simulink model "random_a"  (Simulink 7.1)
settings: Solver=ode45  StartTime=0.0  StopTime=60.0  RelTol=1e-3
settings Model: Creator=Usuario  LastModifiedBy=Usuario  BufferReuse=off
settings OptimizationCC: OptimizeBlockIOStorage=off  BufferReuse=off  ExpressionFolding=off  LocalBlockOutputs=off

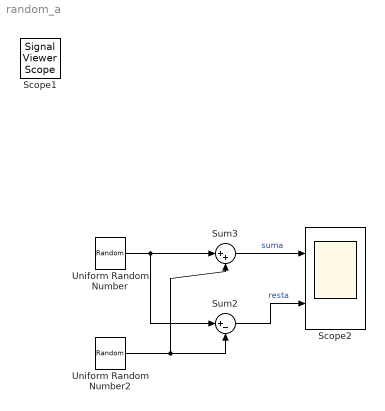
== system random_a ==
  Scope2 : Scope  NumInputPorts=2
      settings: YMin=-5~-5  YMax=5~5  SaveName=ScopeData2
  Sum2 : Sum  Inputs=|+-  OutDataType=sfix(16)  OutScaling=2^0
  Sum3 : Sum  Inputs=|++  OutDataType=sfix(16)  OutScaling=2^0
  Uniform Random Number : UniformRandomNumber  Minimum=0  SampleTime=0
  Uniform Random Number2 : UniformRandomNumber  Minimum=0  Seed=1  SampleTime=0
  Scope1 : SignalViewerScope  IOType=viewer  RefreshTime=0.035000
  wires:
  Uniform Random Number/1 -> Sum3/1, Sum2/1
  Uniform Random Number2/1 -> Sum2/2, Sum3/2
  Sum3/1 -> Scope2/1  "suma"
  Sum2/1 -> Scope2/2  "resta"
